simulink model "paramIden_UKF_friction"  (R2018a)
settings: Solver=ode1  StartTime=0.0  StopTime=20  FixedStep=0.01  RelTol=1e-3
settings Model: Creator=Sarot PC  LastModifiedBy=macuser
settings DataIOCC: SaveFormat=StructureWithTime  ReturnWorkspaceOutputs=on
settings OptimizationCC: LifeSpan=inf
settings DebuggingCC: SFExecutionAtInitializationDiag=none
settings HardwareCC: ProdBitPerSizeT=32  ProdBitPerPtrDiffT=32  ProdWordSize=32  ProdHWDeviceType=Specified
settings SFSimCC: SimUseLocalCustomCode=on
settings RTWCC: RTWUseLocalCustomCode=on
settings CodeAppCC: StateflowObjectComments=on

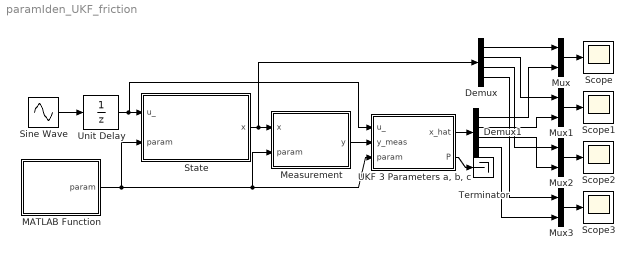
== system paramIden_UKF_friction ==
  Demux : Demux
  Demux1 : Demux
  MATLAB Function : MATLAB Function  TreatAsAtomicUnit=on
  Measurement : MATLAB Function  TreatAsAtomicUnit=on
  Mux{,1..3} (4 alike) : Mux  Inputs=2
  Scope{,1..3} (4 alike) : Scope
  Sine Wave : Sin  Amplitude=10  Bias=2  Frequency=2  SampleTime=0
  State : MATLAB Function  TreatAsAtomicUnit=on
  Terminator : Terminator
  "UKF 3 Parameters a, b, c" : MATLAB Function  TreatAsAtomicUnit=on
  Unit Delay : UnitDelay  SampleTime=0.01
  wires:
  MATLAB Function/1(param) -> State/2(param), Measurement/2(param), "UKF 3 Parameters a, b, c"/3(param)
  State/1(x) -> Demux/1, Measurement/1(x)
  Measurement/1(y) -> "UKF 3 Parameters a, b, c"/2(y_meas)
  "UKF 3 Parameters a, b, c"/2(P) -> Terminator/1
  Demux/1 -> Mux/1
  Demux1/1 -> Mux/2
  Demux/2 -> Mux1/1
  Mux/1 -> Scope/1
  Demux1/2 -> Mux1/2
  Demux/3 -> Mux2/1
  Demux1/3 -> Mux2/2
  Mux1/1 -> Scope1/1
  Mux2/1 -> Scope2/1
  Sine Wave/1 -> Unit Delay/1
  Unit Delay/1 -> "UKF 3 Parameters a, b, c"/1(u_), State/1(u_)
  Mux3/1 -> Scope3/1
  Demux/4 -> Mux3/1
  Demux1/4 -> Mux3/2
  "UKF 3 Parameters a, b, c"/1(x_hat) -> Demux1/1

== matlab function paramIden_UKF_friction/State ==
  settings: updateMethod=DISCRETE
  data: u_ input; x output; param input
function x = fd_true(u_,param)

% w_dot = -a*w + b*u - c*sign(w) + sqrt(Q)*e_s(t) (1)
%                                       (Noise)
% Let x(1)=w, x(2)=a, x(3)=b, x(4)=c, then
% x_dot(1) = -x(1)*x(2) + x(3)*u - x(4)*sign(x(1)) + e1(t)
% x_dot(2) = 0 + e2(t)   (since a is constant)
% x_dot(3) = 0 + e3(t)    (since b is constant)
% x_dot(4) = 0 + e4(t)    (since c is constant)
% In compact form
% x_dot = f(x,u)

% (1) Can be rewritten in discrete form as
% x(k) = x(k-1) + f(x(k-1),u(k-1))*dt + sqrt(dt*Q)*e_s(t)

persistent x_
a = 20; b = 360; c = 270;
if isempty(x_),x_ = [0;a;b;c];end
n = param(1);
dt = param(2);
Q = reshape(param(3:2+n*n),n,n);

x = x_ + [-x_(1)*x_(2)+x_(3)*u_-x_(4)*sigmoidFcn(x_(1));0;0;0]*dt...
    +sqrt(dt)*sqrt(Q)*randn(n,1);
x_= x;
end

function y = sigmoidFcn(x)
y = 2/(1+exp(-20*x))-1;
end

== matlab function paramIden_UKF_friction/MATLAB Function ==
  data: param output
function param = fcn

n  = 4;
m  = 1;
dt = 0.01;

Q = 1e-6*diag([1 10 1 100]);
R = 1e-3;

param = [n;dt;reshape(Q,[],1);m;reshape(R,[],1)];

== matlab function paramIden_UKF_friction/Measurement ==
  data: x input; y output; param input
function y = fcn(x,param)

n = param(1);
m = 1;%param(4+n*n);
R = reshape(param(4+n*n:3+n*n+m*m),m,m);

C = [1 0 0 0];

y = C*x+sqrt(R)*randn(m,1);

== matlab function paramIden_UKF_friction/UKF 3 Parameters a, b, c ==
  settings: updateMethod=DISCRETE
  data: u_ input; x_hat output size=4; P output; y_meas input; param input
function [x_hat,P] = fcn(u_,y_meas,param)

n = param(1);
%dt = param(2);
Q = reshape(param(3:2+n*n),n,n);
m = param(3+n*n);
R = reshape(param(4+n*n:3+n*n+m*m),m,m);

nSigma = 2*n+1;

persistent x_ P_ wm W lambda
if isempty(x_)
    x_= randn(n,1); P_ = 1e-1*eye(n);
    k=2;
    alpha=0.5; beta=1;
    lambda=alpha^2*(n+k)-n;
    Wm0=lambda/(n+lambda);
    Wc0=lambda/((n+lambda)+(1-alpha^2+beta));
    Wmi=1/2/(n+lambda);
    Wci=Wmi;
    wm=Wmi*ones(nSigma,1); wm(1)=Wm0;
    W=(eye(nSigma)-wm*ones(1,nSigma))...
     *diag([Wc0 Wci*ones(1,2*n)])...
     *(eye(nSigma)-wm*ones(1,nSigma))';
end

%Time Update
%Generate Sigma Points
A = chol(P_,'lower');
X_= x_*ones(1,nSigma) + ...
        sqrt(n+lambda)*[zeros(n,1) A -A];
X = X_;
for i=1:nSigma
    X(:,i)= fd(X_(:,i),u_,param);
end
x     = X*wm;
x_hat = x(1:4,1);
P     = X*W*X'+Q+1e-5*diag([1 100 10000 10000]);

%Measurement Update
%Re-Generate Sigma Points
A   = chol(P,'lower');
X   = x*ones(1,nSigma) + ...
        sqrt(n+lambda)*[zeros(n,1) A -A];
Y   = zeros(m,nSigma);
for i=1:nSigma
    Y(:,i)= hd(X(:,i));
end
y   = Y*wm;
Pxy = X*W*Y';
Pyy = Y*W*Y'+R;
K   = Pxy/Pyy;
x_  = x + K*(y_meas-y);
P_  = P - K*Pyy*K';

end

function x = fd(x_,u_,param)
% w_dot = -a*w + b*u - c*sign(w)

% Let x(1)=w, x(2)=a, x(3)=b, x(4)=c, then
% x_dot(1) = -x(1)*x(2) + x(3)*u - x(4)*sign(x(1))
% x_dot(2) = 0    (since a is constant)
% x_dot(3) = 0    (since b is constant)
% x_dot(4) = 0    (since c is constant)
% In compact form
% x_dot = f(x,u)

% Rewritten in discrete form as
% x(k) = x(k-1) + f(x(k-1),u(k-1))*dt

dt = param(2);
x = x_ + [-x_(1)*x_(2)+x_(3)*u_-x_(4)*sigmoidFcn(x_(1));0;0;0]*dt;
end

function y = hd(x)
C = [1 0 0 0];
y = C*x;
end

function y = sigmoidFcn(x)
y = 2/(1+exp(-20*x))-1;
end
